simulink library "Primary_Resistance_StarterV2"  (R2024a)
settings: Solver=VariableStepAuto  StartTime=0.0  StopTime=10.0  RelTol=1e-3
libraries: spsThreePhaseBreakerLib x6, spsThreePhaseParallelRLCBranchLib x4, simulink_extras x1
settings Model: Creator=gshma  LastModifiedBy=gshma

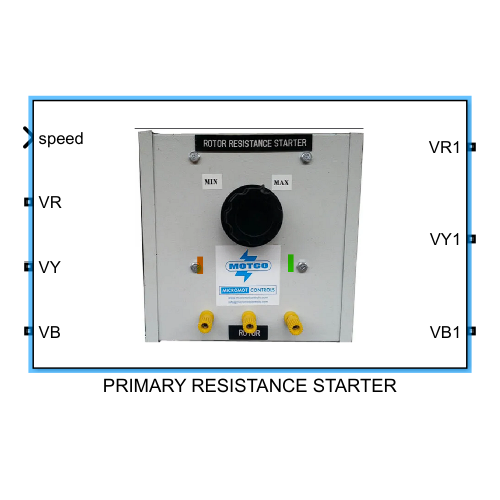
[thumbnail: Simulink's stored preview of the top-level diagram]
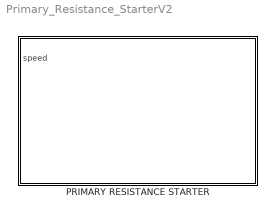
== system Primary_Resistance_StarterV2 ==
  PRIMARY RESISTANCE STARTER : Subsystem
      mask Display: image('pems.png', [0,0,0,0,80,80]);

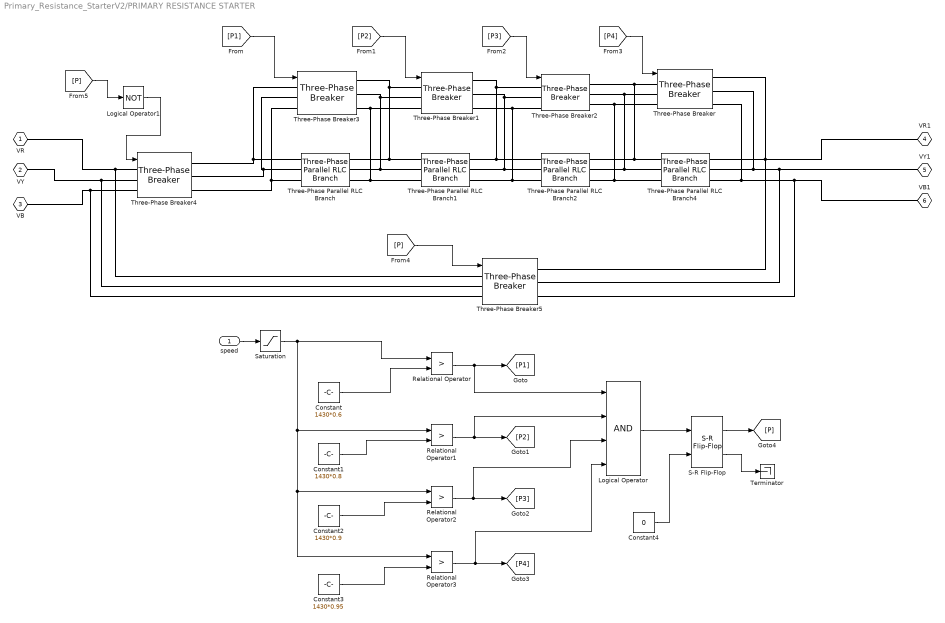
== system Primary_Resistance_StarterV2/PRIMARY RESISTANCE STARTER ==
  speed : Inport
  Constant : Constant  Value=1430*0.6
  Constant1 : Constant  Value=1430*0.8
  Constant2 : Constant  Value=1430*0.9
  Constant3 : Constant  Value=1430*0.95
  Constant4 : Constant  Value=0  OutDataTypeStr=boolean
  Logical Operator : Logic  Inputs=4  AllPortsSameDT=off  OutDataTypeStr=boolean
  Logical Operator1 : Logic  Operator=NOT  AllPortsSameDT=off  OutDataTypeStr=boolean
  Relational Operator{,1..3} (4 alike) : RelationalOperator  Operator=>  OutDataTypeStr=boolean  RndMeth=Simplest  InputSameDT=off
  S-R Flip-Flop : simulink_extras/Flip Flops/S-R Flip-Flop  initial_condition=0
  Saturation : Saturate  UpperLimit=2000  LowerLimit=0
  Terminator : Terminator
  Three-Phase Parallel RLC Branch{,1..2,4} (4 alike) : spsThreePhaseParallelRLCBranchLib/Three-Phase Parallel RLC Branch  LConnTagsString=A|B|C  RConnTagsString=A|B|C  BranchType=R  Resistance=0.8333  Inductance=1e-3  Capacitance=1e-6  Measurements=None
  Three-Phase Breaker{,1..3,5} (5 alike) : spsThreePhaseBreakerLib/Three-Phase Breaker  InitialState=open  SwitchA=on  SwitchB=on  SwitchC=on  SwitchTimes="[1/60  5/60]"  External=on  BreakerResistance=0.01  SnubberResistance=1e6  SnubberCapacitance=inf  Measurements=None
  Three-Phase Breaker4 : spsThreePhaseBreakerLib/Three-Phase Breaker  InitialState=closed  SwitchA=on  SwitchB=on  SwitchC=on  SwitchTimes="[1/60  5/60]"  External=on  BreakerResistance=0.01  SnubberResistance=1e6  SnubberCapacitance=inf  Measurements=None
  VR : PMIOPort  Tag=simrfV2util1/Connection Port  Side=Left
  VY : PMIOPort  Tag=simrfV2util1/Connection Port  Port=2  Side=Left
  VB : PMIOPort  Tag=simrfV2util1/Connection Port  Port=3  Side=Left
  VR1 : PMIOPort  Tag=simrfV2util1/Connection Port  Port=4  Side=Right
  VY1 : PMIOPort  Tag=simrfV2util1/Connection Port  Port=5  Side=Right
  VB1 : PMIOPort  Tag=simrfV2util1/Connection Port  Port=6  Side=Right
  wires:
  Constant/1 -> Relational Operator/2
  Relational Operator/1 -> Logical Operator/1, [P1]
  speed/1 -> Saturation/1
  Relational Operator1/1 -> Logical Operator/2, [P2]
  Constant1/1 -> Relational Operator1/2
  Constant2/1 -> Relational Operator2/2
  Relational Operator2/1 -> Logical Operator/3, [P3]
  Saturation/1 -> Relational Operator3/1, Relational Operator2/1, Relational Operator1/1, Relational Operator/1
  Relational Operator3/1 -> Logical Operator/4, [P4]
  Constant3/1 -> Relational Operator3/2
  [P1] -> Three-Phase Breaker3/1
  [P2] -> Three-Phase Breaker1/1
  [P3] -> Three-Phase Breaker2/1
  [P4] -> Three-Phase Breaker/1
  [P] -> Three-Phase Breaker5/1
  [P] -> Logical Operator1/1
  Logical Operator1/1 -> Three-Phase Breaker4/1
  Logical Operator/1 -> S-R Flip-Flop/1
  S-R Flip-Flop/1 -> [P]
  S-R Flip-Flop/2 -> Terminator/1
  Constant4/1 -> S-R Flip-Flop/2
  connections:
  Three-Phase Parallel RLC Branch/RConn1 -- Three-Phase Breaker1/LConn1 -- Three-Phase Breaker3/RConn1 -- Three-Phase Parallel RLC Branch1/LConn1
  Three-Phase Parallel RLC Branch/RConn2 -- Three-Phase Breaker1/LConn2 -- Three-Phase Breaker3/RConn2 -- Three-Phase Parallel RLC Branch1/LConn2
  Three-Phase Parallel RLC Branch/RConn3 -- Three-Phase Breaker1/LConn3 -- Three-Phase Breaker3/RConn3 -- Three-Phase Parallel RLC Branch1/LConn3
  Three-Phase Parallel RLC Branch1/RConn1 -- Three-Phase Breaker1/RConn1 -- Three-Phase Breaker2/LConn1 -- Three-Phase Parallel RLC Branch2/LConn1
  Three-Phase Parallel RLC Branch1/RConn2 -- Three-Phase Breaker2/LConn2 -- Three-Phase Breaker1/RConn2 -- Three-Phase Parallel RLC Branch2/LConn2
  Three-Phase Parallel RLC Branch1/RConn3 -- Three-Phase Breaker2/LConn3 -- Three-Phase Breaker1/RConn3 -- Three-Phase Parallel RLC Branch2/LConn3
  Three-Phase Parallel RLC Branch2/RConn1 -- Three-Phase Breaker2/RConn1 -- Three-Phase Breaker/LConn1 -- Three-Phase Parallel RLC Branch4/LConn1
  Three-Phase Parallel RLC Branch2/RConn2 -- Three-Phase Breaker2/RConn2 -- Three-Phase Breaker/LConn2 -- Three-Phase Parallel RLC Branch4/LConn2
  Three-Phase Parallel RLC Branch2/RConn3 -- Three-Phase Breaker2/RConn3 -- Three-Phase Breaker/LConn3 -- Three-Phase Parallel RLC Branch4/LConn3
  Three-Phase Breaker3/LConn1 -- Three-Phase Breaker4/RConn1 -- Three-Phase Parallel RLC Branch/LConn1
  Three-Phase Breaker3/LConn2 -- Three-Phase Breaker4/RConn2 -- Three-Phase Parallel RLC Branch/LConn2
  Three-Phase Breaker3/LConn3 -- Three-Phase Breaker4/RConn3 -- Three-Phase Parallel RLC Branch/LConn3
  VR1/RConn1 -- Three-Phase Breaker/RConn1 -- Three-Phase Breaker5/RConn1 -- Three-Phase Parallel RLC Branch4/RConn1
  VY1/RConn1 -- Three-Phase Breaker5/RConn2 -- Three-Phase Breaker/RConn2 -- Three-Phase Parallel RLC Branch4/RConn2
  VB1/RConn1 -- Three-Phase Breaker5/RConn3 -- Three-Phase Breaker/RConn3 -- Three-Phase Parallel RLC Branch4/RConn3
  VR/RConn1 -- Three-Phase Breaker5/LConn1 -- Three-Phase Breaker4/LConn1
  VY/RConn1 -- Three-Phase Breaker5/LConn2 -- Three-Phase Breaker4/LConn2
  VB/RConn1 -- Three-Phase Breaker5/LConn3 -- Three-Phase Breaker4/LConn3
